simulink model "ExampleSensor"  (Simulink 9.2)
settings: Solver=FixedStepDiscrete  StartTime=0.0  StopTime=inf  FixedStep=0.001  RelTol=1e-3  EnableMultiTasking=on
libraries: rFproPhysicsLib x4, simulink x1
Description:
  | Compiled Plugin Only
settings Model: Creator=enewton  LastModifiedBy=SeanKavanagh
settings DataIOCC: LimitDataPoints=off  SaveOutput=off  SignalLogging=off  DSMLogging=off  SaveTime=off
settings DebuggingCC: UnderspecifiedInitializationDetection=Simplified  MergeDetectMultiDrivingBlocksExec=error  StateNameClashWarn=none
settings HardwareCC: ProdIntDivRoundTo=Zero  ProdEndianess=LittleEndian  ProdHWDeviceType=Specified
settings RTWCC: SystemTargetFile=rfpro.tlc  MakeCommand="make_rtw OPTS=\"-DSENSOR\""  TemplateMakefile=rfpro.tmf  Description=rFpro Target (Sensor)  TargetLang=C++
settings STFCustomTargetCC: ModelReferenceCompliant=off  GeneratePreprocessorConditionals=Disable all  CombineOutputUpdateFcns=on  MatFileLogging=on  CPPClassGenCompliant=on  GRTInterface=off  SystemTargetFile=rfpro.tlc
settings GRTTargetCC: ModelReferenceCompliant=off  ParMdlRefBuildCompliant=off  CompOptLevelCompliant=off  ConcurrentExecutionCompliant=off  CombineOutputUpdateFcns=on  GRTInterface=off  UseToolchainInfoCompliant=off

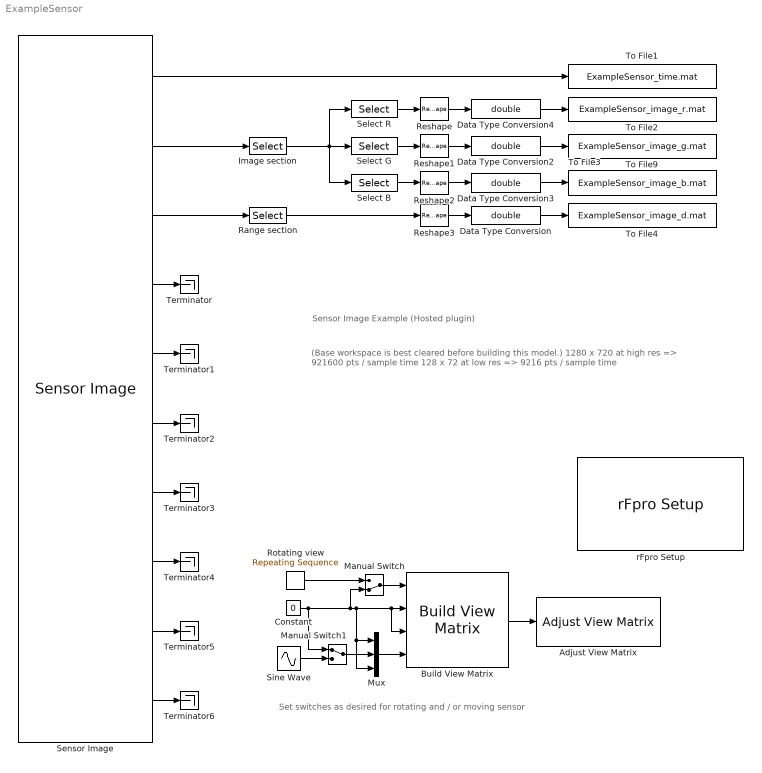
== system ExampleSensor ==
  note: Set switches as desired for rotating and / or moving sensor
  note: Sensor Image Example (Hosted plugin)
  note: (Base workspace is best cleared before building this model.)
      |
      | 1280 x 720 at high res => 921600 pts / sample time
      | 128 x 72 at low res => 9216 pts / sample time
  Adjust View Matrix : rFproPhysicsLib/Hosted Blocks/Adjust View Matrix  SFunctionModules=''
  Build View Matrix : rFproPhysicsLib/Hosted Blocks/Build View Matrix  SystemSampleTime=-1
  Constant : Constant  Value=0
  Data Type Conversion{,2..4} (4 alike) : DataTypeConversion  OutDataTypeStr=double
  Image section : Selector  NumberOfDimensions=3  IndexMode=Zero-based  InputPortWidth=3  IndexOptions=Index vector (dialog),Index vector (dialog),Select all  Indices=[325:396],577:704,1  OutputSizes=72,128,1
  Manual Switch : ManualSwitch  CurrentSetting=0
  Manual Switch1 : ManualSwitch
  Mux : Mux  Inputs=3
  Range section : Selector  NumberOfDimensions=2  IndexMode=Zero-based  InputPortWidth=3  IndexOptions=Index vector (dialog),Index vector (dialog)  Indices=[325:396],577:704  OutputSizes=72,128
  Reshape{,1..3} (4 alike) : Reshape
  Rotating view : simulink/Sources/Repeating Sequence  rep_seq_t=[0 2]  rep_seq_y=[0 2*pi]
  Select B : Selector  NumberOfDimensions=3  IndexMode=Zero-based  InputPortWidth=3  IndexOptions=Select all,Select all,Index vector (dialog)  Indices=[329:392],[569:712],2  OutputSizes=1,1,1
  Select G : Selector  NumberOfDimensions=3  IndexMode=Zero-based  InputPortWidth=3  IndexOptions=Select all,Select all,Index vector (dialog)  Indices=[329:392],[569:712],1  OutputSizes=1,1,1
  Select R : Selector  NumberOfDimensions=3  IndexMode=Zero-based  InputPortWidth=3  IndexOptions=Select all,Select all,Index vector (dialog)  Indices=[329:392],[569:712],0  OutputSizes=1,1,1
  Sensor Image : rFproPhysicsLib/Hosted Blocks/Sensor Image  mode=RGB  range=on  id=off  segmented=off  normal=off  velocity=off  light=off  mat_id=off  fgt=off  format=0  width=1280  height=720  sampleTime=0.001
  Sine Wave : Sin  Amplitude=0.5  Bias=0.5  Frequency=2*pi/2  SampleTime=0
  Terminator{,1..6} (7 alike) : Terminator
  To File1 : ToFile  Filename=ExampleSensor_time.mat  MatrixName=time
  To File2 : ToFile  Filename=ExampleSensor_image_r.mat  MatrixName=red
  To File3 : ToFile  Filename=ExampleSensor_image_b.mat  MatrixName=blue
  To File4 : ToFile  Filename=ExampleSensor_image_d.mat  MatrixName=range
  To File9 : ToFile  Filename=ExampleSensor_image_g.mat  MatrixName=green
  rFpro Setup : rFproPhysicsLib/rFpro Setup  Priority=1  platform=Hosted Plugin  stopOnSessionEnd=on  usePseudoRealtime=on  syncToRF=on  useReverseByteOrder=off  useRfTime=on  minIterations=4  maxIterations=1000  ipReceiveAddress='127.0.0.1'  ipReceivePort=11054  receiveSampleTime=-1  ipTransmitAddress='127.0.0.1'  ipTransmitPort=11052  transmitSampleTime=-1  pluginType=SENSOR
  wires:
  Sensor Image/4 -> Terminator/1
  Sensor Image/5 -> Terminator1/1
  Sensor Image/6 -> Terminator2/1
  Sensor Image/7 -> Terminator3/1
  Reshape1/1 -> Data Type Conversion2/1
  Reshape2/1 -> Data Type Conversion3/1
  Reshape3/1 -> Data Type Conversion/1
  Image section/1 -> Select B/1, Select G/1, Select R/1
  Data Type Conversion4/1 -> To File2/1
  Data Type Conversion2/1 -> To File9/1
  Data Type Conversion3/1 -> To File3/1
  Data Type Conversion/1 -> To File4/1
  Reshape/1 -> Data Type Conversion4/1
  Select R/1 -> Reshape/1
  Select G/1 -> Reshape1/1
  Select B/1 -> Reshape2/1
  Range section/1 -> Reshape3/1
  Build View Matrix/1 -> Adjust View Matrix/1
  Rotating view/1 -> Manual Switch/1
  Constant/1 -> Manual Switch1/1, Manual Switch/2, Build View Matrix/3, Build View Matrix/2, Mux/3, Mux/1
  Sine Wave/1 -> Manual Switch1/2
  Mux/1 -> Build View Matrix/4
  Manual Switch1/1 -> Mux/2
  Manual Switch/1 -> Build View Matrix/1
  Sensor Image/1 -> To File1/1
  Sensor Image/2 -> Image section/1
  Sensor Image/3 -> Range section/1
  Sensor Image/8 -> Terminator4/1
  Sensor Image/9 -> Terminator5/1
  Sensor Image/10 -> Terminator6/1
